simulink model "UAV_2010_simulink_model_run"  (R2023b)
settings: Solver=ode3  StartTime=0.0  StopTime=t_end  FixedStep=1/(8*30)  RelTol=1e-3
values from neighbouring files (symbols this model uses):
  alt0 = 49    [Run_nonlinear_2010UAV_sim.m]
  c_gear = 50    [Run_nonlinear_2010UAV_sim.m]
  gear_deflection_limit = .2    (= 0.2)    [Run_nonlinear_2010UAV_sim.m]
  k_gear = 600    [Run_nonlinear_2010UAV_sim.m]
  lat0 = deg2rad(63.9850)    [Run_nonlinear_2010UAV_sim.m]
  long0 = deg2rad(-22.590)    [Run_nonlinear_2010UAV_sim.m]
  stick_sensitivity = 0.2    [Run_nonlinear_2010UAV_sim.m]
  windseed = [randi([0 4000], 1, 4)]    [Run_nonlinear_2010UAV_sim.m]
  X_init = X_trim_point    [Run_nonlinear_2010UAV_sim.m]
undefined symbols (not defined in the file or in its folder): Applications, F, FlightGear, Light, MIL, Receive, Send
libraries: aerolibfltsims x4, matrix_library x3, aerolibwind2 x2, aerolibatmos2 x1, vrlib x1
settings Model: Creator=aaron  LastModifiedBy=aarongreisen
settings DataIOCC: SaveFormat=StructureWithTime
settings OptimizationCC: ReuseModelBlockBuffer=off
settings DebuggingCC: UnderSpecifiedDimensionMsg=warning

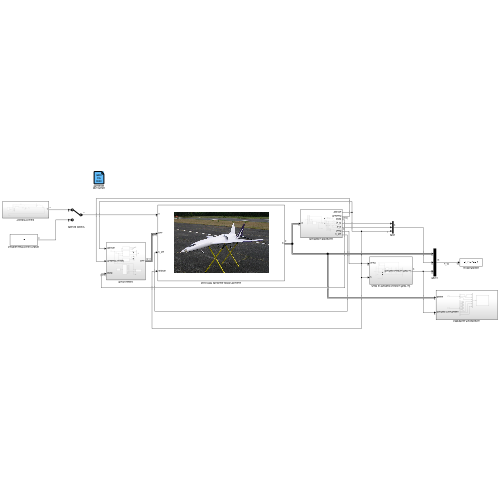
[thumbnail: Simulink's stored preview of the top-level diagram]
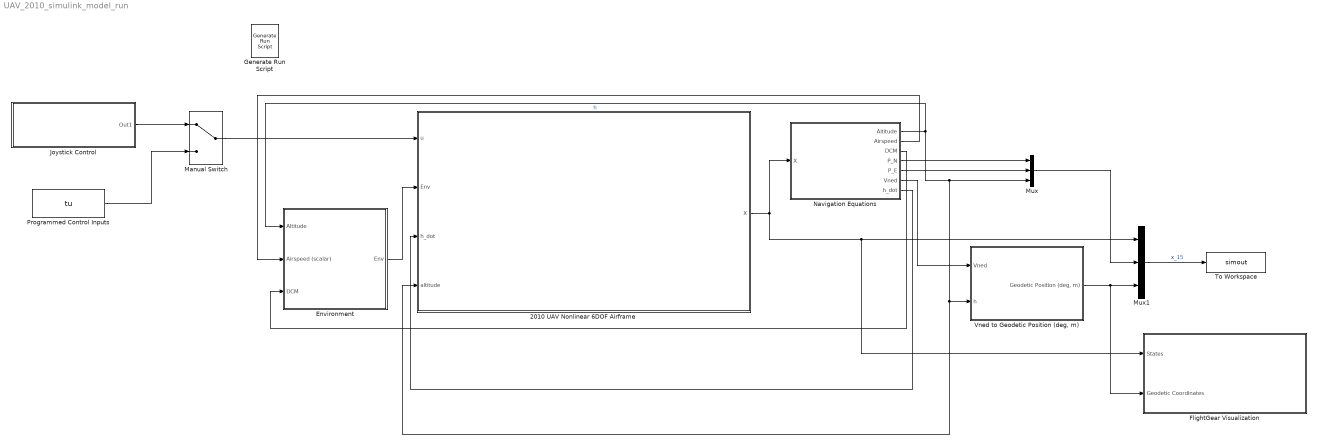
== system UAV_2010_simulink_model_run ==
  2010 UAV Nonlinear 6DOF Airframe : Subsystem
      mask Display: image('$imagefile'); % Use "Edit Image" on toolstrip to change.
  Environment : Subsystem
  FlightGear Visualization : Subsystem
  Generate Run Script : aerolibfltsims/Generate Run Script  Architecture=Mac  dataFlow=Send-Receive  GeometryModelName=c172p  AirportId=KSFO  RunwayId=10L  InitialAltitude=7224  InitialHeading=113  OffsetDistance=4.72  OffsetAzimuth=0  InstallScenery=off  DisableShaders=on  OriginAddress=127.0.0.1  DestinationPort=5502  OriginPort=5505  LocalAddress=127.0.0.1  OutputFileName=fg_simulink_2010UAV.bat  FlightGearBaseDirectory=Applications/FlightGear.app
  Joystick Control : Subsystem
  Manual Switch : ManualSwitch
  Mux : Mux  Inputs=3
  Mux1 : Mux  Inputs=[9 3 3]
  Navigation Equations : Subsystem
  Programmed Control Inputs : FromWorkspace  VariableName=tu
  To Workspace : ToWorkspace  VariableName=simout  SaveFormat=Structure With Time  SampleTime=-1
  "Vned to Geodetic Position (deg, m)" : Subsystem
  wires:
  2010 UAV Nonlinear 6DOF Airframe/1(X) -> Navigation Equations/1(X), Mux1/1, FlightGear Visualization/1(States)
  Navigation Equations/4(P_N) -> Mux/1
  Navigation Equations/5(P_E) -> Mux/2
  Navigation Equations/1(Altitude) -> Environment/1(Altitude), Mux/3, 2010 UAV Nonlinear 6DOF Airframe/4(altitude), "Vned to Geodetic Position (deg, m)"/2(h)  "h"
  Navigation Equations/3(DCM) -> Environment/3(DCM)
  Mux/1 -> Mux1/2
  Mux1/1 -> To Workspace/1  "x_15"
  Navigation Equations/2(Airspeed) -> Environment/2(Airspeed (scalar))
  Navigation Equations/6(Vned) -> "Vned to Geodetic Position (deg, m)"/1(Vned)
  "Vned to Geodetic Position (deg, m)"/1("Geodetic Position (deg, m)") -> FlightGear Visualization/2(Geodetic Coordinates), Mux1/3
  Environment/1(Env) -> 2010 UAV Nonlinear 6DOF Airframe/2(Env)
  Joystick Control/1(Out1) -> Manual Switch/1
  Programmed Control Inputs/1 -> Manual Switch/2
  Manual Switch/1 -> 2010 UAV Nonlinear 6DOF Airframe/1(u)
  Navigation Equations/7(h_dot) -> 2010 UAV Nonlinear 6DOF Airframe/3(h_dot)

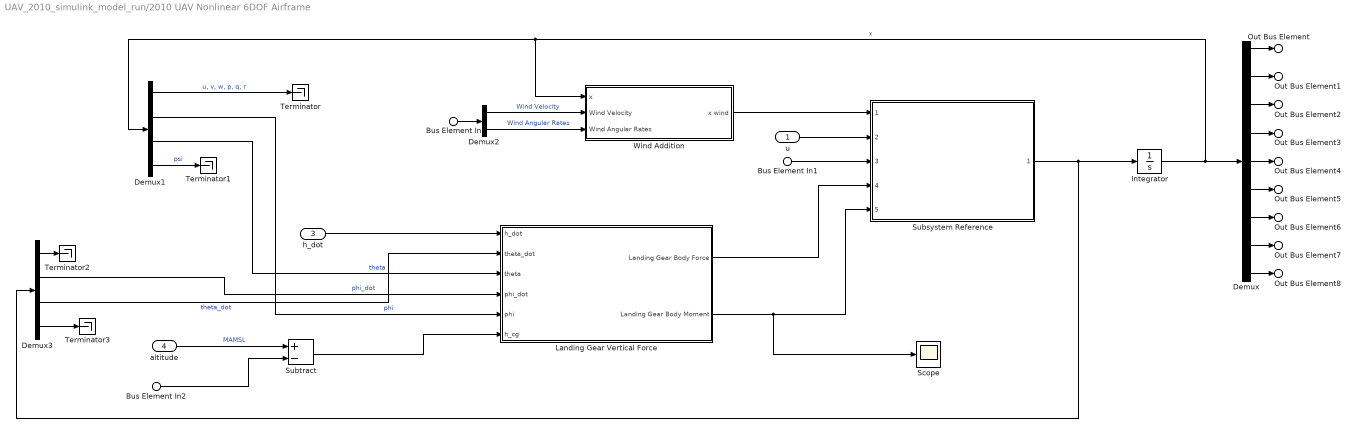
== system UAV_2010_simulink_model_run/2010 UAV Nonlinear 6DOF Airframe ==
  u : Inport
  Bus Element In : Inport  Port=2  PortName=Env  Element=Wind
  Bus Element In1 : Inport  Port=2  PortName=Env  Element=AirDensity
  Bus Element In2 : Inport  Port=2  PortName=Env  Element=hground
  h_dot : Inport  Port=3
  altitude : Inport  Port=4
  Demux : Demux  Outputs=9
  Demux1 : Demux  Outputs=[6 1 1 1]
  Demux2 : Demux  Outputs=[3 3]
  Demux3 : Demux  Outputs=[6 1 1 1]
  Integrator : Integrator  InitialCondition=X_init
  Landing Gear Vertical Force : Subsystem
  Scope : Scope
  Subsystem Reference : Subsystem  ReferencedSubsystem=UAV_2010_Model
  Subtract : Sum  Inputs=+-
  Terminator{,1..3} (4 alike) : Terminator
  Wind Addition : Subsystem
  Out Bus Element : Outport  PortName=X  Element=u
  Out Bus Element1 : Outport  PortName=X  Element=v
  Out Bus Element2 : Outport  PortName=X  Element=w
  Out Bus Element3 : Outport  PortName=X  Element=p
  Out Bus Element4 : Outport  PortName=X  Element=q
  Out Bus Element5 : Outport  PortName=X  Element=r
  Out Bus Element6 : Outport  PortName=X  Element=phi
  Out Bus Element7 : Outport  PortName=X  Element=theta
  Out Bus Element8 : Outport  PortName=X  Element=psi
  wires:
  u/1 -> Subsystem Reference/2
  Integrator/1 -> Wind Addition/1(x), Demux1/1, Demux/1  "x"
  Demux/1 -> Out Bus Element/1
  Demux/2 -> Out Bus Element1/1
  Demux/3 -> Out Bus Element2/1
  Demux/4 -> Out Bus Element3/1
  Demux/5 -> Out Bus Element4/1
  Demux/6 -> Out Bus Element5/1
  Demux/7 -> Out Bus Element6/1
  Demux/8 -> Out Bus Element7/1
  Demux/9 -> Out Bus Element8/1
  Demux2/1 -> Wind Addition/2(Wind Velocity)  "Wind Velocity"
  Demux2/2 -> Wind Addition/3(Wind Angular Rates)  "Wind Angular Rates"
  Wind Addition/1(x wind) -> Subsystem Reference/1
  Bus Element In/1 -> Demux2/1
  Bus Element In1/1 -> Subsystem Reference/3
  h_dot/1 -> Landing Gear Vertical Force/1(h_dot)
  Landing Gear Vertical Force/1(Landing Gear Body Force) -> Subsystem Reference/4
  Landing Gear Vertical Force/2(Landing Gear Body Moment) -> Scope/1, Subsystem Reference/5
  Demux1/1 -> Terminator/1  "u, v, w, p, q, r"
  Demux1/2 -> Landing Gear Vertical Force/5(phi)  "phi"
  Demux1/3 -> Landing Gear Vertical Force/3(theta)  "theta"
  Demux1/4 -> Terminator1/1  "psi"
  Demux3/1 -> Terminator2/1
  Demux3/3 -> Landing Gear Vertical Force/2(theta_dot)  "theta_dot"
  Demux3/2 -> Landing Gear Vertical Force/4(phi_dot)  "phi_dot"
  Demux3/4 -> Terminator3/1
  Subsystem Reference/1 -> Demux3/1, Integrator/1
  Bus Element In2/1 -> Subtract/2
  altitude/1 -> Subtract/1  "MAMSL"
  Subtract/1 -> Landing Gear Vertical Force/6(h_cg)

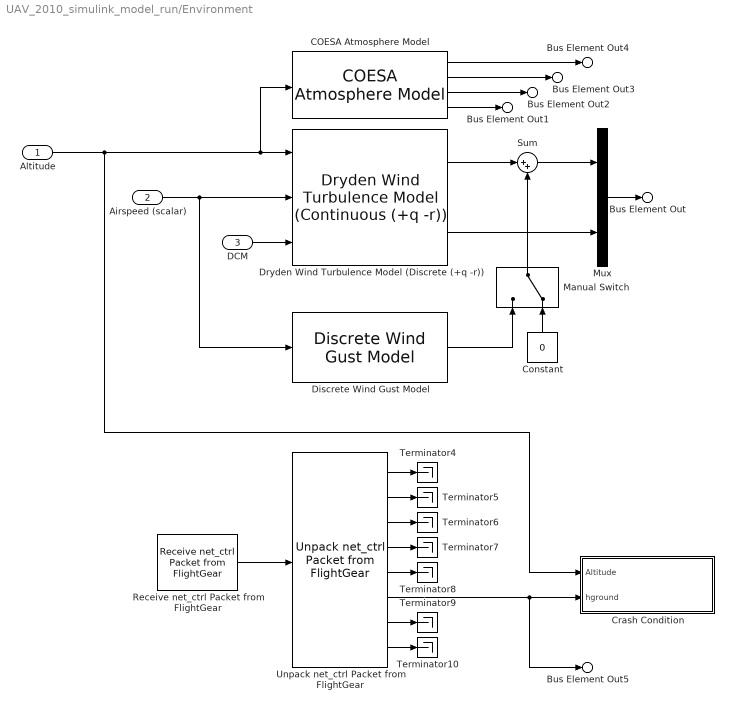
== system UAV_2010_simulink_model_run/Environment ==
  Altitude : Inport
  Airspeed (scalar) : Inport  Port=2
  DCM : Inport  Port=3
  COESA Atmosphere Model : aerolibatmos2/COESA Atmosphere Model  units=Metric (MKS)  spec=1976 COESA-extended U.S. Standard Atmosphere  model=Profile  profile_var=High temperature  profile_percent=1%  profile_alt=5 km (16404 ft)  envelope_var=High temperature  envelope_percent=1%  action=Warning
  Constant : Constant  Value=0
  Crash Condition : Subsystem
  Discrete Wind Gust Model : aerolibwind2/Discrete Wind Gust Model  units=Metric (MKS)  Gx=on  Gy=on  Gz=on  t_0=14  d_m=[120 120 80]  v_m=[3.5 3.5 3.0]
  Dryden Wind Turbulence Model (Discrete (+q -r)) : aerolibwind2/Dryden Wind Turbulence Model  (Continuous (+q -r))  units=Metric (MKS)  spec=MIL-F-8785C  model=Continuous Dryden (+q -r)  W20=3  Wdeg=18  TurbProb=10^-2 - Light  L_high=533.4  Wingspan=1.8657850784  ts=0.1  Seed=windseed  T_on=on
      settings: LibrarySourceBlock=|
      | aerolibwind2/Dryden Wind Turbulence Model
      | (Discrete (+q -r))
  Manual Switch : ManualSwitch  CurrentSetting=0
  Mux : Mux  Inputs=2
  Receive net_ctrl Packet from FlightGear : aerolibfltsims/Receive net_ctrl Packet from FlightGear  FlightGearVersion=v2019.1  ReceiveAddress=127.0.0.1  ReceivePort=5505  ReceiveWidth=744  varLen=off  SampleTime=1/30  packetFlag=off
  Sum : Sum  Inputs=|++
  Terminator{4..10} (7 alike) : Terminator
  Unpack net_ctrl Packet from FlightGear : aerolibfltsims/Unpack net_ctrl Packet from FlightGear  FlightGearVersion=v2019.1  ShowControlSurfacePositionOutputs=off  ShowEngineFuelOutputs=off  ShowLandingGearOutputs=off  ShowAvionicOutputs=off  ShowEnvironmentOutputs=on  SampleTime=1/30  packetVersion=27
  Bus Element Out : Outport  PortName=Env  Element=Wind
  Bus Element Out1 : Outport  PortName=Env  Element=AirDensity
  Bus Element Out2 : Outport  PortName=Env  Element=Air Pressure
  Bus Element Out3 : Outport  PortName=Env  Element=Speed of Sound
  Bus Element Out4 : Outport  PortName=Env  Element=Temperature
  Bus Element Out5 : Outport  PortName=Env  Element=hground
  wires:
  COESA Atmosphere Model/1 -> Bus Element Out4/1
  COESA Atmosphere Model/2 -> Bus Element Out3/1
  COESA Atmosphere Model/3 -> Bus Element Out2/1
  COESA Atmosphere Model/4 -> Bus Element Out1/1
  Dryden Wind Turbulence Model (Discrete (+q -r))/2 -> Mux/2
  Mux/1 -> Bus Element Out/1
  Unpack net_ctrl Packet from FlightGear/5 -> Terminator8/1
  Unpack net_ctrl Packet from FlightGear/8 -> Terminator10/1
  Unpack net_ctrl Packet from FlightGear/2 -> Terminator5/1
  Unpack net_ctrl Packet from FlightGear/6 -> Bus Element Out5/1, Crash Condition/2(hground)
  Unpack net_ctrl Packet from FlightGear/7 -> Terminator9/1
  Unpack net_ctrl Packet from FlightGear/1 -> Terminator4/1
  Unpack net_ctrl Packet from FlightGear/4 -> Terminator7/1
  Receive net_ctrl Packet from FlightGear/1 -> Unpack net_ctrl Packet from FlightGear/1
  Unpack net_ctrl Packet from FlightGear/3 -> Terminator6/1
  Altitude/1 -> Crash Condition/1(Altitude), COESA Atmosphere Model/1, Dryden Wind Turbulence Model (Discrete (+q -r))/1
  Airspeed (scalar)/1 -> Discrete Wind Gust Model/1, Dryden Wind Turbulence Model (Discrete (+q -r))/2
  DCM/1 -> Dryden Wind Turbulence Model (Discrete (+q -r))/3
  Dryden Wind Turbulence Model (Discrete (+q -r))/1 -> Sum/1
  Sum/1 -> Mux/1
  Manual Switch/1 -> Sum/2
  Discrete Wind Gust Model/1 -> Manual Switch/1
  Constant/1 -> Manual Switch/2

== system UAV_2010_simulink_model_run/FlightGear Visualization ==
  States : Inport
  Geodetic Coordinates : Inport  Port=2
  Demux : Demux  Outputs=[1 1 1]
  Demux1 : Demux  Outputs=[1 1 1 1 1 1 1 1 1]
  FlightGear Preconfigured 6DoF Animation : aerolibfltsims/FlightGear Preconfigured 6DoF Animation  xFlightGearVersion=v2019.1  DestinationIpAddress=127.0.0.1  DestinationPort=5502  SampleTime=1/30  packetVersion=24
  Mux2 : Mux  Inputs=[1 1 1 1 1 1]
  Terminator{4..9} (6 alike) : Terminator
  wires:
  States/1 -> Demux1/1
  Demux1/1 -> Terminator4/1
  Demux1/6 -> Terminator9/1
  Demux/2 -> Mux2/1  "Long"
  Demux/3 -> Mux2/3  "Alt"
  Demux1/3 -> Terminator6/1
  Demux1/9 -> Mux2/6  "psi"
  Demux1/4 -> Terminator7/1
  Demux1/7 -> Mux2/4  "phi"
  Demux1/2 -> Terminator5/1
  Demux1/5 -> Terminator8/1
  Mux2/1 -> FlightGear Preconfigured 6DoF Animation/1
  Demux1/8 -> Mux2/5  "theta"
  Demux/1 -> Mux2/2  "Lat"
  Geodetic Coordinates/1 -> Demux/1

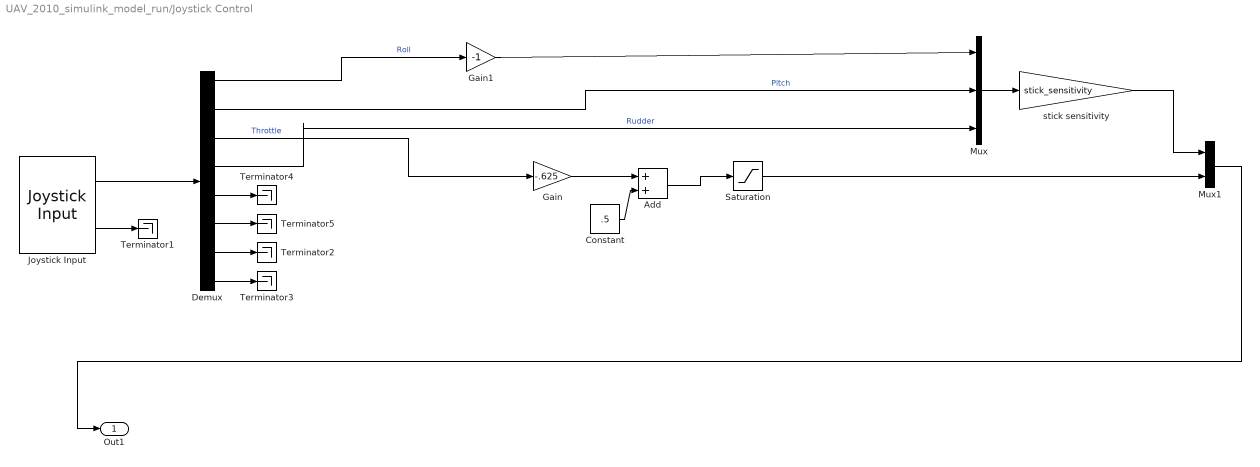
== system UAV_2010_simulink_model_run/Joystick Control ==
  Add : Sum
  Constant : Constant  Value=.5
  Demux : Demux  Outputs=[1 1 1 1 1 1 1 1]
  Gain : Gain  Gain=-.625
  Gain1 : Gain  Gain=-1
  Joystick Input : vrlib/Joystick Input  joyid=1  adjustports=off  forcefeed=off
  Mux : Mux  Inputs=[1 1 1]
  Mux1 : Mux  Inputs=[3 1]
  Saturation : Saturate  UpperLimit=1  LowerLimit=0
  Terminator{1..5} (5 alike) : Terminator
  stick sensitivity : Gain  Gain=stick_sensitivity
  Out1 : Outport
  wires:
  Demux/1 -> Gain1/1  "Roll"
  Saturation/1 -> Mux1/2
  Demux/8 -> Terminator3/1
  Gain/1 -> Add/1
  Joystick Input/1 -> Demux/1
  Add/1 -> Saturation/1
  Demux/4 -> Mux/3  "Rudder"
  Constant/1 -> Add/2
  Demux/7 -> Terminator2/1
  Demux/3 -> Gain/1  "Throttle"
  Mux1/1 -> Out1/1
  Joystick Input/2 -> Terminator1/1
  Demux/5 -> Terminator4/1
  Demux/6 -> Terminator5/1
  Gain1/1 -> Mux/1
  Demux/2 -> Mux/2  "Pitch"
  Mux/1 -> stick sensitivity/1
  stick sensitivity/1 -> Mux1/1

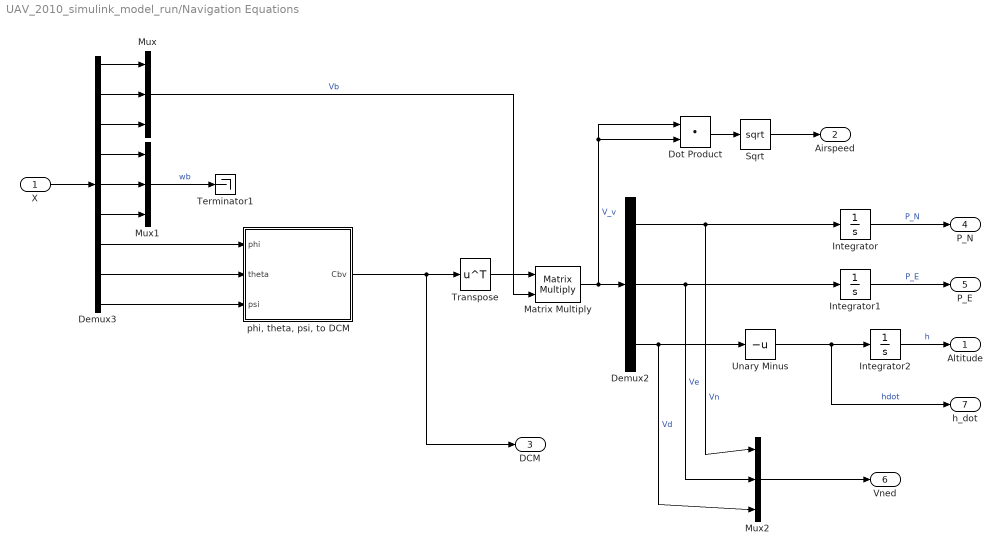
== system UAV_2010_simulink_model_run/Navigation Equations ==
  X : Inport
  Demux2 : Demux  Outputs=3
  Demux3 : Demux  Outputs=9
  Dot Product : DotProduct  OutDataTypeStr=Inherit: Inherit via internal rule
  Integrator : Integrator
  Integrator1 : Integrator
  Integrator2 : Integrator  InitialCondition=alt0
  Matrix Multiply : Product  Multiplication=Matrix(*)
  Mux : Mux  Inputs=3
  Mux1 : Mux  Inputs=3
  Mux2 : Mux  Inputs=[1 1 1]
  Sqrt : Sqrt
  Terminator1 : Terminator
  Transpose : Math  Operator=transpose
  Unary Minus : UnaryMinus
  "phi, theta, psi, to DCM" : MATLAB Function  TreatAsAtomicUnit=on
  Altitude : Outport
  Airspeed : Outport  Port=2
  DCM : Outport  Port=3
  P_N : Outport  Port=4
  P_E : Outport  Port=5
  Vned : Outport  Port=6
  h_dot : Outport  Port=7
  wires:
  Integrator1/1 -> P_E/1  "P_E"
  Demux3/8 -> "phi, theta, psi, to DCM"/2(theta)
  Integrator/1 -> P_N/1  "P_N"
  Matrix Multiply/1 -> Dot Product/1, Dot Product/2, Demux2/1  "V_v"
  Transpose/1 -> Matrix Multiply/1
  Mux/1 -> Matrix Multiply/2  "Vb"
  Mux1/1 -> Terminator1/1  "wb"
  Demux3/7 -> "phi, theta, psi, to DCM"/1(phi)
  Integrator2/1 -> Altitude/1  "h"
  Demux2/2 -> Mux2/2, Integrator1/1  "Ve"
  Demux2/1 -> Mux2/1, Integrator/1  "Vn"
  Demux3/9 -> "phi, theta, psi, to DCM"/3(psi)
  "phi, theta, psi, to DCM"/1(Cbv) -> Transpose/1, DCM/1
  Unary Minus/1 -> h_dot/1, Integrator2/1  "hdot"
  Demux2/3 -> Unary Minus/1, Mux2/3  "Vd"
  X/1 -> Demux3/1
  Demux3/1 -> Mux/1
  Demux3/2 -> Mux/2
  Demux3/3 -> Mux/3
  Demux3/4 -> Mux1/1
  Demux3/5 -> Mux1/2
  Demux3/6 -> Mux1/3
  Dot Product/1 -> Sqrt/1
  Sqrt/1 -> Airspeed/1
  Mux2/1 -> Vned/1

== system UAV_2010_simulink_model_run/Vned to Geodetic Position (deg, m) ==
  Vned : Inport
  h : Inport  Port=2
  Demux : Demux  Outputs=[1 1 1]
  Demux1 : Demux  Outputs=[1 1]
  Gain1 : Gain  Gain=180/pi
  Gain2 : Gain  Gain=180/pi
  Integrator : Integrator  InitialCondition=[lat0 long0]
  Mux : Mux  Inputs=[1 1]
  Mux1 : Mux  Inputs=[1 1 1]
  Terminator : Terminator
  WGS84 Meridian and Prime Vertical Radii : MATLAB Function  TreatAsAtomicUnit=on
  rate of change of latitude : MATLAB Function  TreatAsAtomicUnit=on
  rate of change of longitude : MATLAB Function  TreatAsAtomicUnit=on
  "Geodetic Position (deg, m)" : Outport
  wires:
  Vned/1 -> Demux/1
  Demux/1 -> rate of change of latitude/1(Vn)  "Vn"
  Demux/2 -> rate of change of longitude/1(Ve)  "Ve"
  Mux/1 -> Integrator/1
  rate of change of latitude/1(lat_dot) -> Mux/1  "phi_dot"
  rate of change of longitude/1(long_dot) -> Mux/2  "lambda_dot"
  Integrator/1 -> Demux1/1
  Demux1/2 -> Gain2/1  "longitude (rad)"
  Demux1/1 -> Gain1/1, rate of change of longitude/4(lat), WGS84 Meridian and Prime Vertical Radii/1(lat)  "latitude (rad)"
  Mux1/1 -> "Geodetic Position (deg, m)"/1
  WGS84 Meridian and Prime Vertical Radii/1(M) -> rate of change of latitude/2(M)
  WGS84 Meridian and Prime Vertical Radii/2(N) -> rate of change of longitude/2(N)
  Gain1/1 -> Mux1/1
  Gain2/1 -> Mux1/2
  Demux/3 -> Terminator/1  "Vd"
  h/1 -> Mux1/3, rate of change of latitude/3(h), rate of change of longitude/3(h)

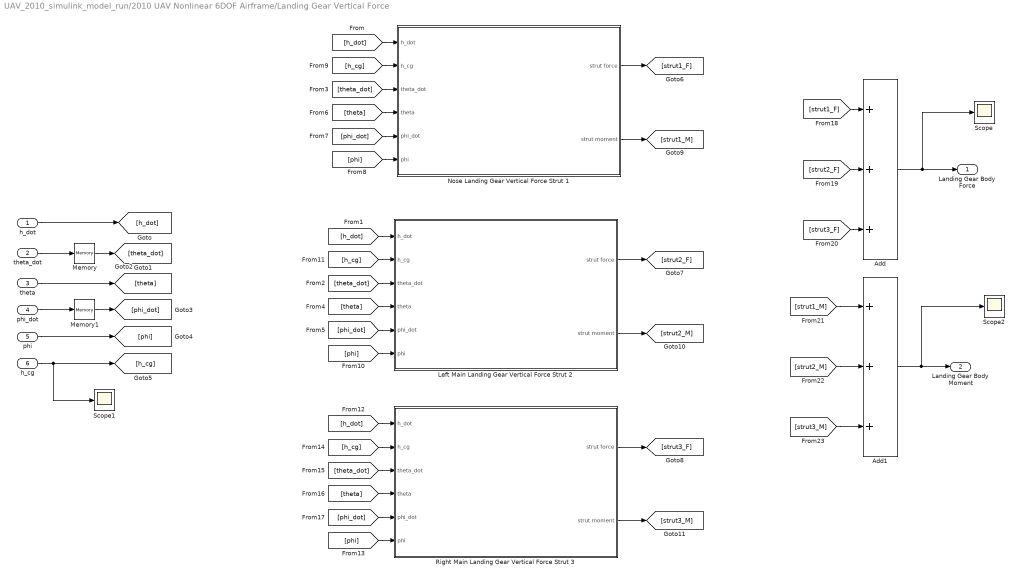
== system UAV_2010_simulink_model_run/2010 UAV Nonlinear 6DOF Airframe/Landing Gear Vertical Force ==
  h_dot : Inport
  theta_dot : Inport  Port=2
  theta : Inport  Port=3
  phi_dot : Inport  Port=4
  phi : Inport  Port=5
  h_cg : Inport  Port=6
  Add : Sum  Inputs=+++
  Add1 : Sum  Inputs=+++
  Left Main Landing Gear Vertical Force Strut 2 : Subsystem
  Memory : Memory
  Memory1 : Memory
  Nose Landing Gear Vertical Force Strut 1 : Subsystem
  Right Main Landing Gear Vertical Force Strut 3 : Subsystem
  Scope : Scope
  Scope1 : Scope
  Scope2 : Scope
  Landing Gear Body Force : Outport
  Landing Gear Body Moment : Outport  Port=2
  wires:
  theta_dot/1 -> Memory/1
  phi_dot/1 -> Memory1/1
  Add/1 -> Scope/1, Landing Gear Body Force/1
  Add1/1 -> Scope2/1, Landing Gear Body Moment/1
  h_dot/1 -> [h_dot]
  [h_dot] -> Nose Landing Gear Vertical Force Strut 1/1(h_dot)
  Memory/1 -> [theta_dot]
  [theta_dot] -> Nose Landing Gear Vertical Force Strut 1/3(theta_dot)
  theta/1 -> [theta]
  [theta] -> Nose Landing Gear Vertical Force Strut 1/4(theta)
  Memory1/1 -> [phi_dot]
  phi/1 -> [phi]
  h_cg/1 -> Scope1/1, [h_cg]
  [phi_dot] -> Nose Landing Gear Vertical Force Strut 1/5(phi_dot)
  [phi] -> Nose Landing Gear Vertical Force Strut 1/6(phi)
  [h_cg] -> Nose Landing Gear Vertical Force Strut 1/2(h_cg)
  Nose Landing Gear Vertical Force Strut 1/1(strut force) -> [strut1_F]
  Left Main Landing Gear Vertical Force Strut 2/1(strut force) -> [strut2_F]
  Right Main Landing Gear Vertical Force Strut 3/1(strut force) -> [strut3_F]
  [strut1_F] -> Add/1
  [strut2_F] -> Add/2
  [strut3_F] -> Add/3
  Nose Landing Gear Vertical Force Strut 1/2(strut moment) -> [strut1_M]
  Left Main Landing Gear Vertical Force Strut 2/2(strut moment) -> [strut2_M]
  Right Main Landing Gear Vertical Force Strut 3/2(strut moment) -> [strut3_M]
  [strut1_M] -> Add1/1
  [strut2_M] -> Add1/2
  [strut3_M] -> Add1/3
  [h_dot] -> Left Main Landing Gear Vertical Force Strut 2/1(h_dot)
  [theta_dot] -> Left Main Landing Gear Vertical Force Strut 2/3(theta_dot)
  [theta] -> Left Main Landing Gear Vertical Force Strut 2/4(theta)
  [phi_dot] -> Left Main Landing Gear Vertical Force Strut 2/5(phi_dot)
  [phi] -> Left Main Landing Gear Vertical Force Strut 2/6(phi)
  [h_cg] -> Left Main Landing Gear Vertical Force Strut 2/2(h_cg)
  [h_dot] -> Right Main Landing Gear Vertical Force Strut 3/1(h_dot)
  [theta] -> Right Main Landing Gear Vertical Force Strut 3/4(theta)
  [phi] -> Right Main Landing Gear Vertical Force Strut 3/6(phi)
  [phi_dot] -> Right Main Landing Gear Vertical Force Strut 3/5(phi_dot)
  [theta_dot] -> Right Main Landing Gear Vertical Force Strut 3/3(theta_dot)
  [h_cg] -> Right Main Landing Gear Vertical Force Strut 3/2(h_cg)

== system UAV_2010_simulink_model_run/2010 UAV Nonlinear 6DOF Airframe/Wind Addition ==
  x : Inport
  Wind Velocity : Inport  Port=2
  Wind Angular Rates : Inport  Port=3
  Demux1 : Demux  Outputs=[1 1 1 1 1 1 1 1 1]
  Mux1 : Mux  Inputs=[1 1 1]
  Mux2 : Mux  Inputs=[1 1 1]
  Mux3 : Mux  Inputs=[6, 3]
  Mux4 : Mux  Inputs=[1 1 1]
  Mux5 : Mux  Inputs=[3 3]
  Sum : Sum  Inputs=|+-
  Sum1 : Sum  Inputs=|++
  x wind : Outport
  wires:
  Sum/1 -> Mux5/1
  Demux1/1 -> Mux2/1  "u"
  Demux1/3 -> Mux2/3  "w"
  Mux4/1 -> Sum1/1
  Demux1/4 -> Mux4/1  "p"
  Wind Angular Rates/1 -> Sum1/2
  Mux2/1 -> Sum/1
  Demux1/7 -> Mux1/1  "phi"
  Demux1/6 -> Mux4/3  "r"
  Demux1/5 -> Mux4/2  "q"
  Mux1/1 -> Mux3/2
  Demux1/2 -> Mux2/2  "v"
  Demux1/9 -> Mux1/3  "psi"
  Sum1/1 -> Mux5/2
  Mux5/1 -> Mux3/1
  Demux1/8 -> Mux1/2  "theta"
  Wind Velocity/1 -> Sum/2
  x/1 -> Demux1/1
  Mux3/1 -> x wind/1

== system UAV_2010_simulink_model_run/Environment/Crash Condition ==
  Altitude : Inport
  hground : Inport  Port=2
  Assertion : Assertion  AssertionFailFcn="disp(\"Airplane Crashed\")"  StopWhenAssertionFail=off
  Constant : Constant  Value=0
  LessThanOrEqual : RelationalOperator  Operator=<=  OutDataTypeStr=boolean  RndMeth=Simplest  InputSameDT=off
  Minus : Sum  Inputs=+-
  NOT : Logic  Operator=NOT  IconShape=distinctive  AllPortsSameDT=off  OutDataTypeStr=boolean
  Stop Simulation : Stop
  wires:
  Minus/1 -> LessThanOrEqual/1
  Altitude/1 -> Minus/1
  Constant/1 -> LessThanOrEqual/2
  hground/1 -> Minus/2
  LessThanOrEqual/1 -> NOT/1, Stop Simulation/1
  NOT/1 -> Assertion/1

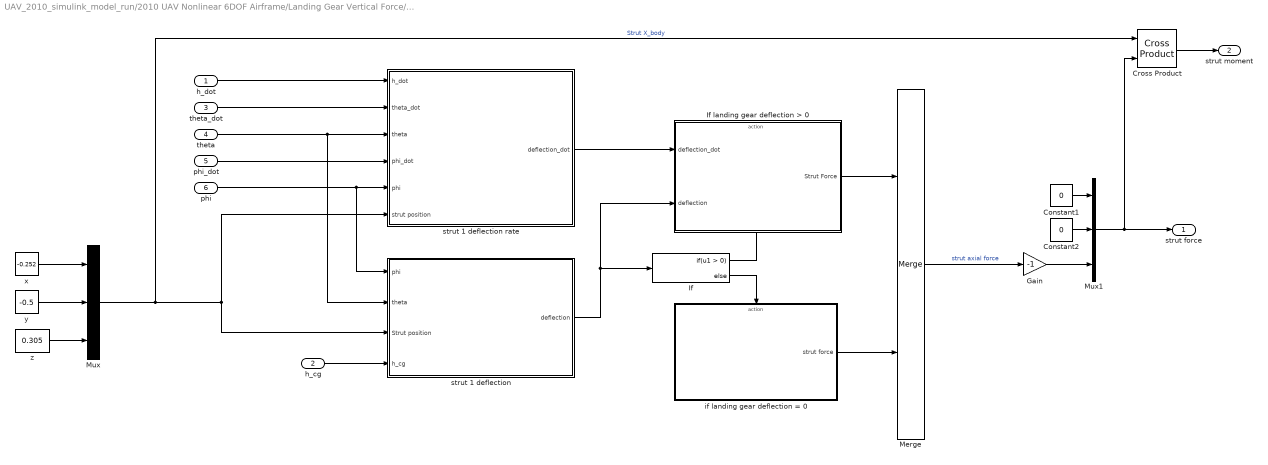
== system UAV_2010_simulink_model_run/2010 UAV Nonlinear 6DOF Airframe/Landing Gear Vertical Force/Left Main Landing Gear Vertical Force Strut 2 ==
  h_dot : Inport
  h_cg : Inport  Port=2
  theta_dot : Inport  Port=3
  theta : Inport  Port=4
  phi_dot : Inport  Port=5
  phi : Inport  Port=6
  Constant1 : Constant  Value=0
  Constant2 : Constant  Value=0
  Cross Product : matrix_library/Cross Product
  Gain : Gain  Gain=-1
  If : If
  If landing gear deflection > 0 : Subsystem  TreatAsAtomicUnit=on
  Merge : Merge
  Mux : Mux  Inputs=[1 1 1]
  Mux1 : Mux  Inputs=[1 1 1]
  if landing gear deflection = 0 : Subsystem  TreatAsAtomicUnit=on
  strut 1 deflection : Subsystem
  strut 1 deflection rate : Subsystem
  x : Constant  Value=-0.252
  y : Constant  Value=-0.5
  z : Constant  Value=0.305
  strut force : Outport
  strut moment : Outport  Port=2
  wires:
  if landing gear deflection = 0/1(strut force) -> Merge/2
  If/1 -> If landing gear deflection > 0/Action
  If/2 -> if landing gear deflection = 0/Action
  If landing gear deflection > 0/1(Strut Force) -> Merge/1
  Merge/1 -> Gain/1  "strut axial force"
  strut 1 deflection/1(deflection) -> If landing gear deflection > 0/2(deflection), If/1
  h_dot/1 -> strut 1 deflection rate/1(h_dot)
  theta_dot/1 -> strut 1 deflection rate/2(theta_dot)
  theta/1 -> strut 1 deflection rate/3(theta), strut 1 deflection/2(theta)
  phi_dot/1 -> strut 1 deflection rate/4(phi_dot)
  phi/1 -> strut 1 deflection rate/5(phi), strut 1 deflection/1(phi)
  h_cg/1 -> strut 1 deflection/4(h_cg)
  z/1 -> Mux/3
  x/1 -> Mux/1
  Mux/1 -> strut 1 deflection/3(Strut position), strut 1 deflection rate/6(strut position), Cross Product/1  "Strut X_body"
  Constant1/1 -> Mux1/1
  Constant2/1 -> Mux1/2
  Mux1/1 -> strut force/1, Cross Product/2
  Cross Product/1 -> strut moment/1
  Gain/1 -> Mux1/3
  strut 1 deflection rate/1(deflection_dot) -> If landing gear deflection > 0/1(deflection_dot)
  y/1 -> Mux/2

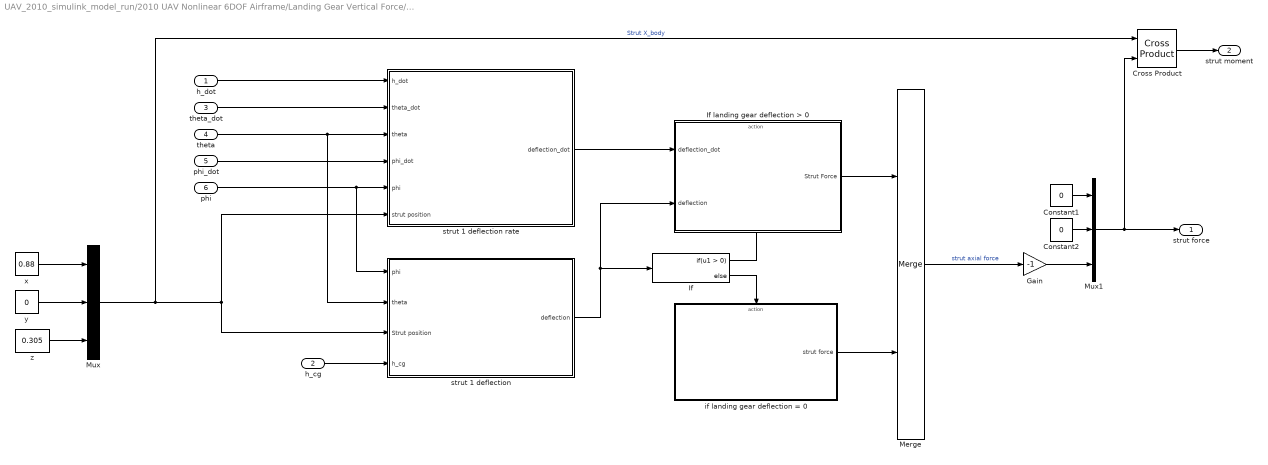
== system UAV_2010_simulink_model_run/2010 UAV Nonlinear 6DOF Airframe/Landing Gear Vertical Force/Nose Landing Gear Vertical Force Strut 1 ==
  h_dot : Inport
  h_cg : Inport  Port=2
  theta_dot : Inport  Port=3
  theta : Inport  Port=4
  phi_dot : Inport  Port=5
  phi : Inport  Port=6
  Constant1 : Constant  Value=0
  Constant2 : Constant  Value=0
  Cross Product : matrix_library/Cross Product
  Gain : Gain  Gain=-1
  If : If
  If landing gear deflection > 0 : Subsystem  TreatAsAtomicUnit=on
  Merge : Merge
  Mux : Mux  Inputs=[1 1 1]
  Mux1 : Mux  Inputs=[1 1 1]
  if landing gear deflection = 0 : Subsystem  TreatAsAtomicUnit=on
  strut 1 deflection : Subsystem
  strut 1 deflection rate : Subsystem
  x : Constant  Value=0.88
  y : Constant  Value=0
  z : Constant  Value=0.305
  strut force : Outport
  strut moment : Outport  Port=2
  wires:
  if landing gear deflection = 0/1(strut force) -> Merge/2
  If/1 -> If landing gear deflection > 0/Action
  If/2 -> if landing gear deflection = 0/Action
  If landing gear deflection > 0/1(Strut Force) -> Merge/1
  Merge/1 -> Gain/1  "strut axial force"
  strut 1 deflection/1(deflection) -> If landing gear deflection > 0/2(deflection), If/1
  h_dot/1 -> strut 1 deflection rate/1(h_dot)
  theta_dot/1 -> strut 1 deflection rate/2(theta_dot)
  theta/1 -> strut 1 deflection rate/3(theta), strut 1 deflection/2(theta)
  phi_dot/1 -> strut 1 deflection rate/4(phi_dot)
  phi/1 -> strut 1 deflection rate/5(phi), strut 1 deflection/1(phi)
  h_cg/1 -> strut 1 deflection/4(h_cg)
  z/1 -> Mux/3
  x/1 -> Mux/1
  Mux/1 -> strut 1 deflection/3(Strut position), strut 1 deflection rate/6(strut position), Cross Product/1  "Strut X_body"
  Constant1/1 -> Mux1/1
  Constant2/1 -> Mux1/2
  Mux1/1 -> strut force/1, Cross Product/2
  Cross Product/1 -> strut moment/1
  Gain/1 -> Mux1/3
  strut 1 deflection rate/1(deflection_dot) -> If landing gear deflection > 0/1(deflection_dot)
  y/1 -> Mux/2

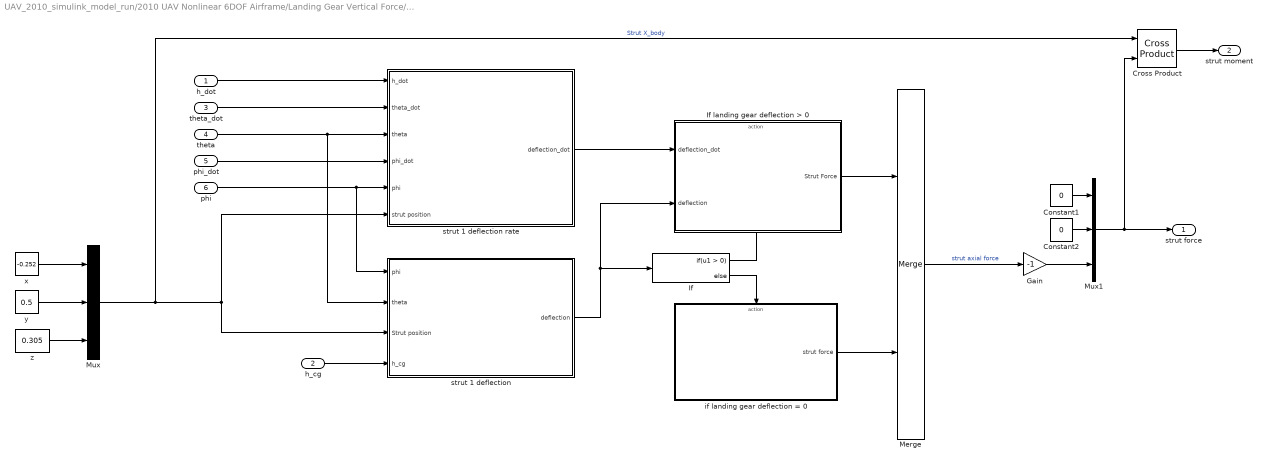
== system UAV_2010_simulink_model_run/2010 UAV Nonlinear 6DOF Airframe/Landing Gear Vertical Force/Right Main Landing Gear Vertical Force Strut 3 ==
  h_dot : Inport
  h_cg : Inport  Port=2
  theta_dot : Inport  Port=3
  theta : Inport  Port=4
  phi_dot : Inport  Port=5
  phi : Inport  Port=6
  Constant1 : Constant  Value=0
  Constant2 : Constant  Value=0
  Cross Product : matrix_library/Cross Product
  Gain : Gain  Gain=-1
  If : If
  If landing gear deflection > 0 : Subsystem  TreatAsAtomicUnit=on
  Merge : Merge
  Mux : Mux  Inputs=[1 1 1]
  Mux1 : Mux  Inputs=[1 1 1]
  if landing gear deflection = 0 : Subsystem  TreatAsAtomicUnit=on
  strut 1 deflection : Subsystem
  strut 1 deflection rate : Subsystem
  x : Constant  Value=-0.252
  y : Constant  Value=0.5
  z : Constant  Value=0.305
  strut force : Outport
  strut moment : Outport  Port=2
  wires:
  if landing gear deflection = 0/1(strut force) -> Merge/2
  If/1 -> If landing gear deflection > 0/Action
  If/2 -> if landing gear deflection = 0/Action
  If landing gear deflection > 0/1(Strut Force) -> Merge/1
  Merge/1 -> Gain/1  "strut axial force"
  strut 1 deflection/1(deflection) -> If landing gear deflection > 0/2(deflection), If/1
  h_dot/1 -> strut 1 deflection rate/1(h_dot)
  theta_dot/1 -> strut 1 deflection rate/2(theta_dot)
  theta/1 -> strut 1 deflection rate/3(theta), strut 1 deflection/2(theta)
  phi_dot/1 -> strut 1 deflection rate/4(phi_dot)
  phi/1 -> strut 1 deflection rate/5(phi), strut 1 deflection/1(phi)
  h_cg/1 -> strut 1 deflection/4(h_cg)
  z/1 -> Mux/3
  x/1 -> Mux/1
  Mux/1 -> strut 1 deflection/3(Strut position), strut 1 deflection rate/6(strut position), Cross Product/1  "Strut X_body"
  Constant1/1 -> Mux1/1
  Constant2/1 -> Mux1/2
  Mux1/1 -> strut force/1, Cross Product/2
  Cross Product/1 -> strut moment/1
  Gain/1 -> Mux1/3
  strut 1 deflection rate/1(deflection_dot) -> If landing gear deflection > 0/1(deflection_dot)
  y/1 -> Mux/2

== system UAV_2010_simulink_model_run/2010 UAV Nonlinear 6DOF Airframe/Landing Gear Vertical Force/Left Main Landing Gear Vertical Force Strut 2/If landing gear deflection > 0 ==
  deflection_dot : Inport
  deflection : Inport  Port=2
  Action Port : ActionPort  ActionPortLabel=if(u1 > 0)
  Add : Sum
  Product : Product
  Product1 : Product
  c : Constant  Value=c_gear
  k : Constant  Value=k_gear
  Strut Force : Outport
  wires:
  deflection_dot/1 -> Product/1
  c/1 -> Product/2
  deflection/1 -> Product1/1
  k/1 -> Product1/2
  Product/1 -> Add/1
  Product1/1 -> Add/2
  Add/1 -> Strut Force/1

== system UAV_2010_simulink_model_run/2010 UAV Nonlinear 6DOF Airframe/Landing Gear Vertical Force/Left Main Landing Gear Vertical Force Strut 2/if landing gear deflection = 0 ==
  Action Port : ActionPort  ActionPortLabel=else
  zero : Constant  Value=0
  strut force : Outport
  wires:
  zero/1 -> strut force/1

== system UAV_2010_simulink_model_run/2010 UAV Nonlinear 6DOF Airframe/Landing Gear Vertical Force/Left Main Landing Gear Vertical Force Strut 2/strut 1 deflection ==
  note: The landing gear deflection is $\delta_t = z_i - h_{c.g.}-x_i\sin\theta+y_i\sin\phi$ where $[x_i, y_i, z_i]$ are the coordinates of the wheel with respect to the cg.
  note: X
  note: y
  note: z
  phi : Inport
  theta : Inport  Port=2
  Strut position : Inport  Port=3
  h_cg : Inport  Port=4
  Add : Sum
  Demux : Demux  Outputs=[1 1 1]
  Product : Product
  Product1 : Product
  Saturation : Saturate  UpperLimit=gear_deflection_limit  LowerLimit=0
  Sin : Trigonometry
  Sin1 : Trigonometry
  Subtract : Sum  Inputs=+-
  Subtract1 : Sum  Inputs=-+
  deflection : Outport
  wires:
  theta/1 -> Sin/1
  Sin/1 -> Product/2  "sin(theta)"
  Sin1/1 -> Product1/2  "sin(theta)"
  phi/1 -> Sin1/1
  Demux/3 -> Subtract/1  "strut z"
  Strut position/1 -> Demux/1
  Saturation/1 -> deflection/1
  h_cg/1 -> Subtract/2
  Subtract/1 -> Add/2
  Demux/1 -> Product/1  "strut x"
  Demux/2 -> Product1/1  "strut y"
  Product1/1 -> Add/1
  Add/1 -> Subtract1/2  "deflection"
  Product/1 -> Subtract1/1
  Subtract1/1 -> Saturation/1

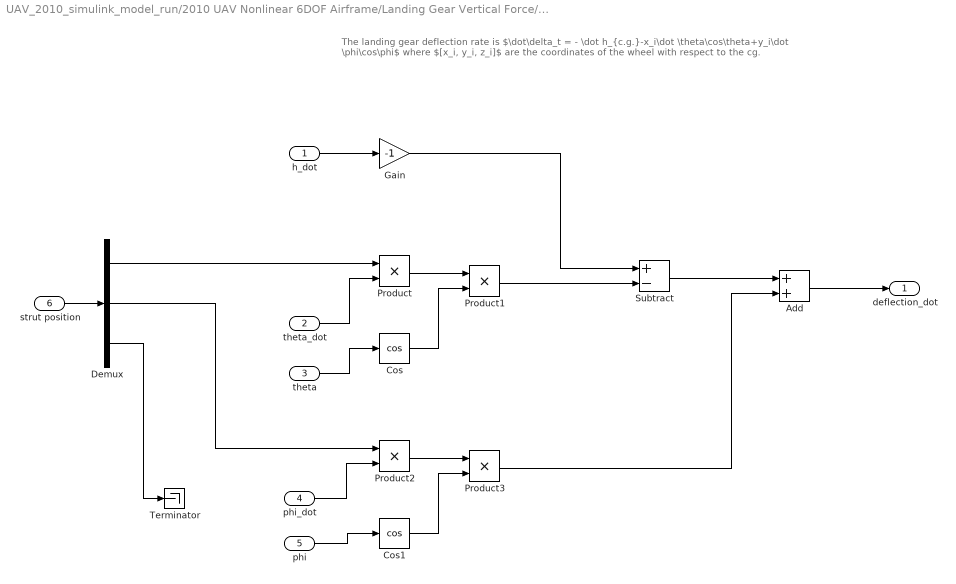
== system UAV_2010_simulink_model_run/2010 UAV Nonlinear 6DOF Airframe/Landing Gear Vertical Force/Left Main Landing Gear Vertical Force Strut 2/strut 1 deflection rate ==
  note: The landing gear deflection rate is $\dot\delta_t = - \dot h_{c.g.}-x_i\dot \theta\cos\theta+y_i\dot \phi\cos\phi$ where $[x_i, y_i, z_i]$ are the coordinates of the wheel with respect to the cg.
  h_dot : Inport
  theta_dot : Inport  Port=2
  theta : Inport  Port=3
  phi_dot : Inport  Port=4
  phi : Inport  Port=5
  strut position : Inport  Port=6
  Add : Sum
  Cos : Trigonometry  Operator=cos
  Cos1 : Trigonometry  Operator=cos
  Demux : Demux  Outputs=[1 1 1]
  Gain : Gain  Gain=-1
  Product{,1..3} (4 alike) : Product
  Subtract : Sum  Inputs=+-
  Terminator : Terminator
  deflection_dot : Outport
  wires:
  h_dot/1 -> Gain/1
  Demux/1 -> Product/1
  theta_dot/1 -> Product/2
  theta/1 -> Cos/1
  Product1/1 -> Subtract/2
  Product/1 -> Product1/1
  Cos/1 -> Product1/2
  Gain/1 -> Subtract/1
  Product2/1 -> Product3/1
  Cos1/1 -> Product3/2
  Demux/2 -> Product2/1
  phi_dot/1 -> Product2/2
  phi/1 -> Cos1/1
  Subtract/1 -> Add/1
  Product3/1 -> Add/2
  Add/1 -> deflection_dot/1
  strut position/1 -> Demux/1
  Demux/3 -> Terminator/1

== system UAV_2010_simulink_model_run/2010 UAV Nonlinear 6DOF Airframe/Landing Gear Vertical Force/Nose Landing Gear Vertical Force Strut 1/If landing gear deflection > 0 ==
  deflection_dot : Inport
  deflection : Inport  Port=2
  Action Port : ActionPort  ActionPortLabel=if(u1 > 0)
  Add : Sum
  Product : Product
  Product1 : Product
  c : Constant  Value=c_gear
  k : Constant  Value=k_gear
  Strut Force : Outport
  wires:
  deflection_dot/1 -> Product/1
  c/1 -> Product/2
  deflection/1 -> Product1/1
  k/1 -> Product1/2
  Product/1 -> Add/1
  Product1/1 -> Add/2
  Add/1 -> Strut Force/1

== system UAV_2010_simulink_model_run/2010 UAV Nonlinear 6DOF Airframe/Landing Gear Vertical Force/Nose Landing Gear Vertical Force Strut 1/if landing gear deflection = 0 ==
  Action Port : ActionPort  ActionPortLabel=else
  zero : Constant  Value=0
  strut force : Outport
  wires:
  zero/1 -> strut force/1

== system UAV_2010_simulink_model_run/2010 UAV Nonlinear 6DOF Airframe/Landing Gear Vertical Force/Nose Landing Gear Vertical Force Strut 1/strut 1 deflection ==
  note: The landing gear deflection is modelled using $\delta_t = z_i - h_{c.g.}-x_i\sin\theta+y_i\sin\phi$ where $[x_i, y_i, z_i]$ are the coordinates of the wheel with respect to the cg.
  note: X
  note: y
  note: z
  phi : Inport
  theta : Inport  Port=2
  Strut position : Inport  Port=3
  h_cg : Inport  Port=4
  Add : Sum
  Demux : Demux  Outputs=[1 1 1]
  Product : Product
  Product1 : Product
  Saturation : Saturate  UpperLimit=gear_deflection_limit  LowerLimit=0
  Sin : Trigonometry
  Sin1 : Trigonometry
  Subtract : Sum  Inputs=+-
  Subtract1 : Sum  Inputs=-+
  deflection : Outport
  wires:
  theta/1 -> Sin/1
  Sin/1 -> Product/2  "sin(theta)"
  Sin1/1 -> Product1/2  "sin(theta)"
  phi/1 -> Sin1/1
  Demux/3 -> Subtract/1  "strut z"
  Strut position/1 -> Demux/1
  Saturation/1 -> deflection/1
  h_cg/1 -> Subtract/2
  Subtract/1 -> Add/2
  Demux/1 -> Product/1  "strut x"
  Demux/2 -> Product1/1  "strut y"
  Product1/1 -> Add/1
  Add/1 -> Subtract1/2  "deflection"
  Product/1 -> Subtract1/1
  Subtract1/1 -> Saturation/1

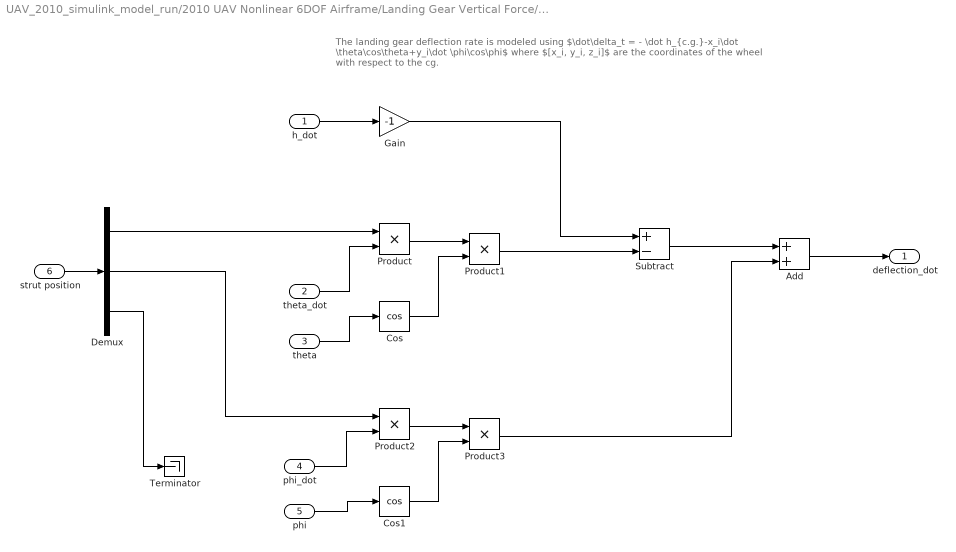
== system UAV_2010_simulink_model_run/2010 UAV Nonlinear 6DOF Airframe/Landing Gear Vertical Force/Nose Landing Gear Vertical Force Strut 1/strut 1 deflection rate ==
  note: The landing gear deflection rate is modeled using $\dot\delta_t = - \dot h_{c.g.}-x_i\dot \theta\cos\theta+y_i\dot \phi\cos\phi$ where $[x_i, y_i, z_i]$ are the coordinates of the wheel with respect to the cg.
  h_dot : Inport
  theta_dot : Inport  Port=2
  theta : Inport  Port=3
  phi_dot : Inport  Port=4
  phi : Inport  Port=5
  strut position : Inport  Port=6
  Add : Sum
  Cos : Trigonometry  Operator=cos
  Cos1 : Trigonometry  Operator=cos
  Demux : Demux  Outputs=[1 1 1]
  Gain : Gain  Gain=-1
  Product{,1..3} (4 alike) : Product
  Subtract : Sum  Inputs=+-
  Terminator : Terminator
  deflection_dot : Outport
  wires:
  h_dot/1 -> Gain/1
  Demux/1 -> Product/1
  theta_dot/1 -> Product/2
  theta/1 -> Cos/1
  Product1/1 -> Subtract/2
  Product/1 -> Product1/1
  Cos/1 -> Product1/2
  Gain/1 -> Subtract/1
  Product2/1 -> Product3/1
  Cos1/1 -> Product3/2
  Demux/2 -> Product2/1
  phi_dot/1 -> Product2/2
  phi/1 -> Cos1/1
  Subtract/1 -> Add/1
  Product3/1 -> Add/2
  Add/1 -> deflection_dot/1
  strut position/1 -> Demux/1
  Demux/3 -> Terminator/1

== system UAV_2010_simulink_model_run/2010 UAV Nonlinear 6DOF Airframe/Landing Gear Vertical Force/Right Main Landing Gear Vertical Force Strut 3/If landing gear deflection > 0 ==
  deflection_dot : Inport
  deflection : Inport  Port=2
  Action Port : ActionPort  ActionPortLabel=if(u1 > 0)
  Add : Sum
  Product : Product
  Product1 : Product
  c : Constant  Value=c_gear
  k : Constant  Value=k_gear
  Strut Force : Outport
  wires:
  deflection_dot/1 -> Product/1
  c/1 -> Product/2
  deflection/1 -> Product1/1
  k/1 -> Product1/2
  Product/1 -> Add/1
  Product1/1 -> Add/2
  Add/1 -> Strut Force/1

== system UAV_2010_simulink_model_run/2010 UAV Nonlinear 6DOF Airframe/Landing Gear Vertical Force/Right Main Landing Gear Vertical Force Strut 3/if landing gear deflection = 0 ==
  Action Port : ActionPort  ActionPortLabel=else
  zero : Constant  Value=0
  strut force : Outport
  wires:
  zero/1 -> strut force/1

== system UAV_2010_simulink_model_run/2010 UAV Nonlinear 6DOF Airframe/Landing Gear Vertical Force/Right Main Landing Gear Vertical Force Strut 3/strut 1 deflection ==
  note: The landing gear deflection is $\delta_t = z_i - h_{c.g.}-x_i\sin\theta+y_i\sin\phi$ where $[x_i, y_i, z_i]$ are the coordinates of the wheel with respect to the cg.
  note: X
  note: y
  note: z
  phi : Inport
  theta : Inport  Port=2
  Strut position : Inport  Port=3
  h_cg : Inport  Port=4
  Add : Sum
  Demux : Demux  Outputs=[1 1 1]
  Product : Product
  Product1 : Product
  Saturation : Saturate  UpperLimit=gear_deflection_limit  LowerLimit=0
  Sin : Trigonometry
  Sin1 : Trigonometry
  Subtract : Sum  Inputs=+-
  Subtract1 : Sum  Inputs=-+
  deflection : Outport
  wires:
  theta/1 -> Sin/1
  Sin/1 -> Product/2  "sin(theta)"
  Sin1/1 -> Product1/2  "sin(theta)"
  phi/1 -> Sin1/1
  Demux/3 -> Subtract/1  "strut z"
  Strut position/1 -> Demux/1
  Saturation/1 -> deflection/1
  h_cg/1 -> Subtract/2
  Subtract/1 -> Add/2
  Demux/1 -> Product/1  "strut x"
  Demux/2 -> Product1/1  "strut y"
  Product1/1 -> Add/1
  Add/1 -> Subtract1/2  "deflection"
  Product/1 -> Subtract1/1
  Subtract1/1 -> Saturation/1

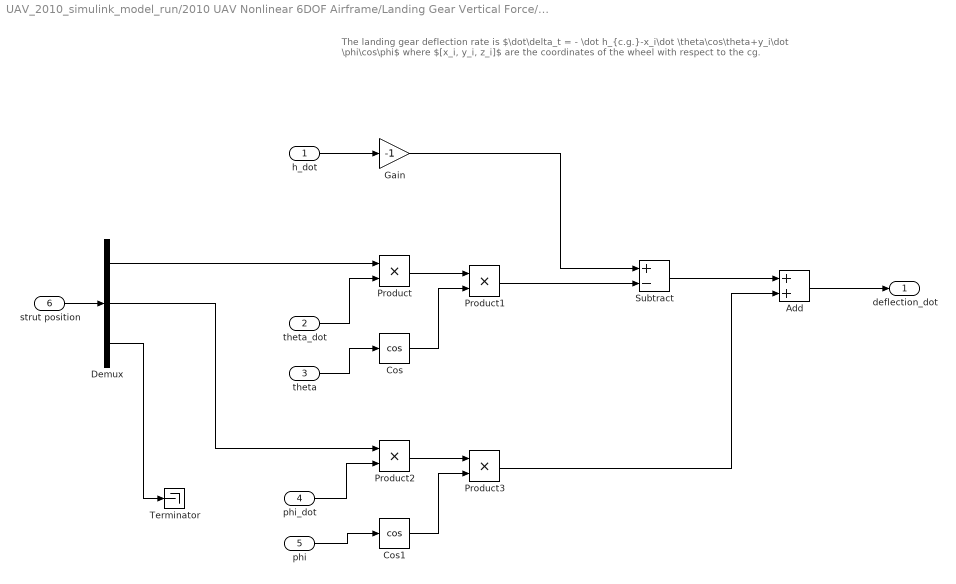
== system UAV_2010_simulink_model_run/2010 UAV Nonlinear 6DOF Airframe/Landing Gear Vertical Force/Right Main Landing Gear Vertical Force Strut 3/strut 1 deflection rate ==
  note: The landing gear deflection rate is $\dot\delta_t = - \dot h_{c.g.}-x_i\dot \theta\cos\theta+y_i\dot \phi\cos\phi$ where $[x_i, y_i, z_i]$ are the coordinates of the wheel with respect to the cg.
  h_dot : Inport
  theta_dot : Inport  Port=2
  theta : Inport  Port=3
  phi_dot : Inport  Port=4
  phi : Inport  Port=5
  strut position : Inport  Port=6
  Add : Sum
  Cos : Trigonometry  Operator=cos
  Cos1 : Trigonometry  Operator=cos
  Demux : Demux  Outputs=[1 1 1]
  Gain : Gain  Gain=-1
  Product{,1..3} (4 alike) : Product
  Subtract : Sum  Inputs=+-
  Terminator : Terminator
  deflection_dot : Outport
  wires:
  h_dot/1 -> Gain/1
  Demux/1 -> Product/1
  theta_dot/1 -> Product/2
  theta/1 -> Cos/1
  Product1/1 -> Subtract/2
  Product/1 -> Product1/1
  Cos/1 -> Product1/2
  Gain/1 -> Subtract/1
  Product2/1 -> Product3/1
  Cos1/1 -> Product3/2
  Demux/2 -> Product2/1
  phi_dot/1 -> Product2/2
  phi/1 -> Cos1/1
  Subtract/1 -> Add/1
  Product3/1 -> Add/2
  Add/1 -> deflection_dot/1
  strut position/1 -> Demux/1
  Demux/3 -> Terminator/1

== matlab function UAV_2010_simulink_model_run/Vned to Geodetic Position (deg, m)/WGS84 Meridian and Prime Vertical Radii ==
  data: lat input; M output; N output
function [M, N] = meridian_curvature(lat)

a = 6378137.0;
e = 0.081819190842622;

M = a*(1-e^2)/(1 - e^2*sin(lat)^2)^(3/2);
N = a/(1 - e^2*sin(lat)^2)^(1/2);

== matlab function UAV_2010_simulink_model_run/Navigation Equations/phi, theta, psi, to DCM ==
  data: phi input; Cbv output; theta input; psi input
function Cbv = calc_Cbv(phi, theta, psi)

C1v = [ cos(psi) sin(psi)  0
       -sin(psi) cos(psi)  0
        0        0         1];

C21 = [cos(theta)  0  -sin(theta)
       0           1   0
       sin(theta)  0   cos(theta)];

Cb2 = [1  0        0
       0  cos(phi) sin(phi)
       0 -sin(phi) cos(phi)];

Cbv = Cb2*C21*C1v;

== matlab function UAV_2010_simulink_model_run/Vned to Geodetic Position (deg, m)/rate of change of latitude ==
  data: Vn input; lat_dot output; M input; h input
function lat_dot = latitude_rate(Vn, M, h)

lat_dot = Vn/(M+h);

== matlab function UAV_2010_simulink_model_run/Vned to Geodetic Position (deg, m)/rate of change of longitude ==
  data: Ve input; long_dot output; N input; h input; lat input
function long_dot = longitude_rate(Ve, N, h, lat)

long_dot = Ve/((N+h)*cos(lat));
